simulink model "vj2_simulink"  (R2020b)
settings: Solver=VariableStepAuto  StartTime=0.0  StopTime=120  RelTol=1e-3
values from neighbouring files (symbols this model uses):
  A = [0 1;0 -D/J]    [vj2.m]
  B = [0;i/J]    [vj2.m]
  C = [1 0;0 1]    [vj2.m]
  Kd = 35    [vj2.m]
  Ki = 0    [vj2.m]
  Kp = 35    [vj2.m]
settings Model: Creator=dominik  LastModifiedBy=dominik
settings DataIOCC: ReturnWorkspaceOutputs=off

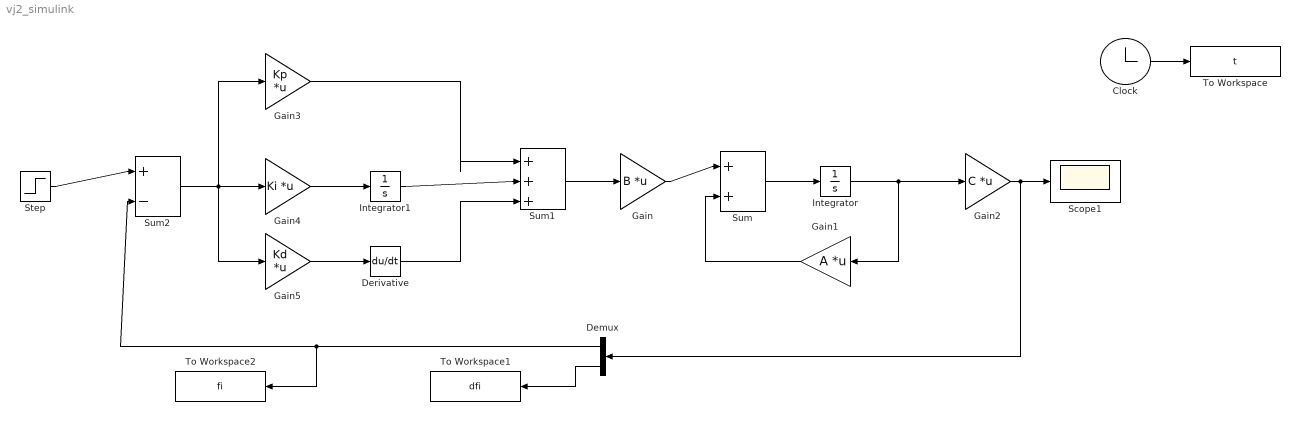
== system vj2_simulink ==
  Clock : Clock
  Demux : Demux  Outputs=2
  Derivative : Derivative
  Gain : Gain  Gain=B  Multiplication=Matrix(K*u)
  Gain1 : Gain  Gain=A  Multiplication=Matrix(K*u)
  Gain2 : Gain  Gain=C  Multiplication=Matrix(K*u)
  Gain3 : Gain  Gain=Kp  Multiplication=Matrix(K*u)
  Gain4 : Gain  Gain=Ki  Multiplication=Matrix(K*u)
  Gain5 : Gain  Gain=Kd  Multiplication=Matrix(K*u)
  Integrator : Integrator
  Integrator1 : Integrator
  Scope1 : Scope
  Step : Step  After=u  SampleTime=0
  Sum : Sum  Inputs=|++
  Sum1 : Sum  Inputs=|+++
  Sum2 : Sum  Inputs=|+-
  To Workspace : ToWorkspace  VariableName=t  SaveFormat=Timeseries  SampleTime=-1
  To Workspace1 : ToWorkspace  VariableName=dfi  SampleTime=-1
      settings: Save2DSignal=2-D array (concatenate along first dimension)
  To Workspace2 : ToWorkspace  VariableName=fi  SampleTime=-1
      settings: Save2DSignal=2-D array (concatenate along first dimension)
  wires:
  Gain/1 -> Sum/1
  Sum/1 -> Integrator/1
  Gain1/1 -> Sum/2
  Integrator/1 -> Gain2/1, Gain1/1
  Gain2/1 -> Demux/1, Scope1/1
  Sum1/1 -> Gain/1
  Derivative/1 -> Sum1/3
  Integrator1/1 -> Sum1/2
  Gain3/1 -> Sum1/1
  Gain4/1 -> Integrator1/1
  Gain5/1 -> Derivative/1
  Sum2/1 -> Gain5/1, Gain3/1, Gain4/1
  Step/1 -> Sum2/1
  Demux/1 -> To Workspace2/1, Sum2/2
  Clock/1 -> To Workspace/1
  Demux/2 -> To Workspace1/1
